simulink model "FAdder"  (Simulink 7.1)
settings: Solver=VariableStepDiscrete  StartTime=0.0  StopTime=10.0  RelTol=1e-3
settings Model: Creator=temp  LastModifiedBy=subramanian.krishnan
settings SolverCC: AutoInsertRateTranBlk=on
settings DebuggingCC: SaveWithParameterizedLinksMsg=none  SolverPrmCheckMsg=none  InheritedTsInSrcMsg=none  DiscreteInheritContinuousMsg=none  TasksWithSamePriorityMsg=none  SigSpecEnsureSampleTimeMsg=none
settings GRTTargetCC: TargetFcnLib=ansi_tfl_tmw.mat

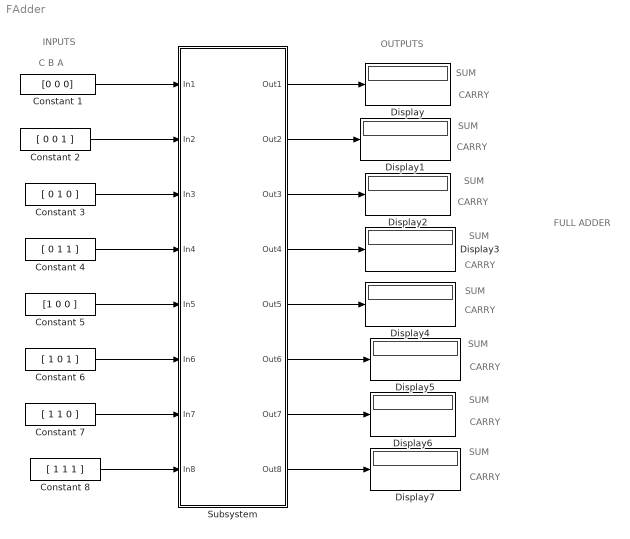
== system FAdder ==
  note: FULL ADDER
  note: SUM
  note: CARRY
  note: SUM
  note: CARRY
  note: SUM
  note: CARRY
  note: SUM
  note: CARRY
  note: SUM
  note: CARRY
  note: SUM
  note: CARRY
  note: SUM
  note: CARRY
  note: SUM
  note: CARRY
  note: OUTPUTS
  note: INPUTS
  note: C B A
  Constant 1 : Constant  Value=[0 0 0]  OutDataTypeMode=boolean  OutDataType=sfix(16)  OutScaling=2^0  OutDataTypeStr=boolean
  Constant 2 : Constant  Value=[ 0 0 1 ]  OutDataTypeMode=boolean  OutDataType=sfix(16)  OutScaling=2^0  OutDataTypeStr=boolean
  Constant 3 : Constant  Value=[ 0 1 0 ]  OutDataTypeMode=boolean  OutDataType=sfix(16)  OutScaling=2^0  OutDataTypeStr=boolean
  Constant 4 : Constant  Value=[ 0 1 1 ]  OutDataTypeMode=boolean  OutDataType=sfix(16)  OutScaling=2^0  OutDataTypeStr=boolean
  Constant 5 : Constant  Value=[1 0 0 ]  OutDataTypeMode=boolean  OutDataType=sfix(16)  OutScaling=2^0  OutDataTypeStr=boolean
  Constant 6 : Constant  Value=[ 1 0 1 ]  OutDataTypeMode=boolean  OutDataType=sfix(16)  OutScaling=2^0  OutDataTypeStr=boolean
  Constant 7 : Constant  Value=[ 1 1 0 ]  OutDataTypeMode=boolean  OutDataType=sfix(16)  OutScaling=2^0  OutDataTypeStr=boolean
  Constant 8 : Constant  Value=[ 1 1 1 ]  OutDataTypeMode=boolean  OutDataType=sfix(16)  OutScaling=2^0  OutDataTypeStr=boolean
  Display{,1..7} (8 alike) : Display
  Subsystem : Subsystem
  wires:
  Constant 1/1 -> Subsystem/1(In1)
  Constant 2/1 -> Subsystem/2(In2)
  Constant 3/1 -> Subsystem/3(In3)
  Constant 4/1 -> Subsystem/4(In4)
  Constant 5/1 -> Subsystem/5(In5)
  Constant 6/1 -> Subsystem/6(In6)
  Constant 7/1 -> Subsystem/7(In7)
  Constant 8/1 -> Subsystem/8(In8)
  Subsystem/1(Out1) -> Display/1
  Subsystem/2(Out2) -> Display1/1
  Subsystem/3(Out3) -> Display2/1
  Subsystem/4(Out4) -> Display3/1
  Subsystem/5(Out5) -> Display4/1
  Subsystem/6(Out6) -> Display5/1
  Subsystem/7(Out7) -> Display6/1
  Subsystem/8(Out8) -> Display7/1

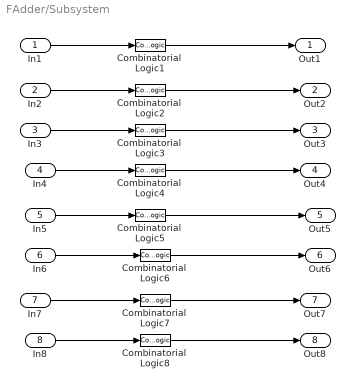
== system FAdder/Subsystem ==
  In1 : Inport  DataType=boolean  OutDataType=sfix(16)  OutScaling=2^0  OutDataTypeStr=boolean
  In2 : Inport  Port=2  DataType=boolean  OutDataType=sfix(16)  OutScaling=2^0  OutDataTypeStr=boolean
  In3 : Inport  Port=3  DataType=boolean  OutDataType=sfix(16)  OutScaling=2^0  OutDataTypeStr=boolean
  In4 : Inport  Port=4  DataType=boolean  OutDataType=sfix(16)  OutScaling=2^0  OutDataTypeStr=boolean
  In5 : Inport  Port=5  DataType=boolean  OutDataType=sfix(16)  OutScaling=2^0  OutDataTypeStr=boolean
  In6 : Inport  Port=6  DataType=boolean  OutDataType=sfix(16)  OutScaling=2^0  OutDataTypeStr=boolean
  In7 : Inport  Port=7  DataType=boolean  OutDataType=sfix(16)  OutScaling=2^0  OutDataTypeStr=boolean
  In8 : Inport  Port=8  DataType=boolean  OutDataType=sfix(16)  OutScaling=2^0  OutDataTypeStr=boolean
  Combinatorial  Logic{1..8} (8 alike) : CombinatorialLogic  TruthTable=[0 0;1 0 ;1 0;0 1;1 0;0 1;0 1;1 1]
  Out1 : Outport  DataType=boolean  OutDataType=sfix(16)  OutScaling=2^0  OutDataTypeStr=boolean
  Out2 : Outport  Port=2  DataType=boolean  OutDataType=sfix(16)  OutScaling=2^0  OutDataTypeStr=boolean
  Out3 : Outport  Port=3  DataType=boolean  OutDataType=sfix(16)  OutScaling=2^0  OutDataTypeStr=boolean
  Out4 : Outport  Port=4  DataType=boolean  OutDataType=sfix(16)  OutScaling=2^0  OutDataTypeStr=boolean
  Out5 : Outport  Port=5  DataType=boolean  OutDataType=sfix(16)  OutScaling=2^0  OutDataTypeStr=boolean
  Out6 : Outport  Port=6  DataType=boolean  OutDataType=sfix(16)  OutScaling=2^0  OutDataTypeStr=boolean
  Out7 : Outport  Port=7  DataType=boolean  OutDataType=sfix(16)  OutScaling=2^0  OutDataTypeStr=boolean
  Out8 : Outport  Port=8  DataType=boolean  OutDataType=sfix(16)  OutScaling=2^0  OutDataTypeStr=boolean
  wires:
  In1/1 -> Combinatorial  Logic1/1
  Combinatorial  Logic1/1 -> Out1/1
  In2/1 -> Combinatorial  Logic2/1
  In3/1 -> Combinatorial  Logic3/1
  In4/1 -> Combinatorial  Logic4/1
  In5/1 -> Combinatorial  Logic5/1
  In6/1 -> Combinatorial  Logic6/1
  In7/1 -> Combinatorial  Logic7/1
  In8/1 -> Combinatorial  Logic8/1
  Combinatorial  Logic2/1 -> Out2/1
  Combinatorial  Logic3/1 -> Out3/1
  Combinatorial  Logic4/1 -> Out4/1
  Combinatorial  Logic5/1 -> Out5/1
  Combinatorial  Logic6/1 -> Out6/1
  Combinatorial  Logic7/1 -> Out7/1
  Combinatorial  Logic8/1 -> Out8/1
